simulink model "TJA1042_Loop_Example"  (R2024a)
(part 4 of 5)

      | CanConfigSet/CanController_0/CanCpuClockRef - /Mcu/Mcu/McuModuleConfiguration/McuClockSettingConfig_0/FLEXCAN_PE_CLK0_2 
      | CanConfigSet/CanController_0/CanCpuClockRefAlternate - /Mcu/Mcu/McuModuleConfiguration/McuClockSettingConfig_0/FLEXCAN_PE_CLK0_2 
      | CanConfigSet/CanController_0/CanHwChannel - FLEXCAN_0 
      | CanConfigSet/CanController_0/CanLoopBackMode - false 
      | CanConfigSet/CanController_0/CanRamBlock - CanRamBlock 
      | CanConfigSet/CanController_0/CanRamBlock/CanRamBlockUnified - CanRamBlockUnified 
      | CanConfigSet/CanController_0/CanRamBlock/CanRamBlockUnified/CanBlockUnifiedPayloadLength - CAN_16_BYTES_PAYLOAD 
      | CanConfigSet/CanController_0/CanRamBlock/Choice - CanRamBlockUnified 
      | CanConfigSet/CanController_0/CanRamBlock/Index - 0 
      | CanConfigSet/CanController_0/CanRxFiFo - CanRxFiFo 
      | CanConfigSet/CanController_0/CanRxFiFo/CanEnhanceFiFo - CanRxFiFo 
      | CanConfigSet/CanController_0/CanRxFiFo/CanRxFiFo/CanEnhanceFiFoDmaEnable - false 
      | CanConfigSet/CanController_0/CanRxFiFo/CanRxFiFo/CanEnhancedSchemeType - MASK_FILTER_SCHEME 
      | CanConfigSet/CanController_0/CanRxFiFo/CanRxFiFo/CanFiFoDmaErrorNotif - NULL_PTR 
      | CanConfigSet/CanController_0/CanRxFiFo/CanRxFiFo/CanFiFoOverflowNotif - MBDT_FlexCAN0_FifoOverflowNotif 
      | CanConfigSet/CanController_0/CanRxFiFo/CanRxFiFo/NumberMBTransferDMA - 1 
      | CanConfigSet/CanController_0/CanRxFiFo/Choice - CanEnhanceFiFo 
      | CanConfigSet/CanController_0/CanRxFiFo/Index - 0 
      | CanConfigSet/CanController_0/CanRxProcessing - MIXED 
      | CanConfigSet/CanController_0/CanTrippleSamplingEnable - false 
      | CanConfigSet/CanController_0/CanTxProcessing - MIXED 
      | CanConfigSet/CanController_0/CanWakeupFunctionalityAPI - false 
      | CanConfigSet/CanController_0/CanWakeupProcessing - POLLING 
      | CanConfigSet/CanController_0/CanWakeupSupport - false 
      | CanConfigSet/CanController_0/Index - 0 
      | CanConfigSet/CanController_1/CanAutoBusOffRecovery - false 
      | CanConfigSet/CanController_1/CanBusoffProcessing - POLLING 
      | CanConfigSet/CanController_1/CanControllerActivation - true 
      | CanConfigSet/CanController_1/CanControllerBaseAddress - 0 
      | CanConfigSet/CanController_1/CanControllerBaudrateConfig - CanControllerBaudrateConfig_0 
      | CanConfigSet/CanController_1/CanControllerBaudrateConfig_0/CanAdvancedSetting - false 
      | CanConfigSet/CanController_1/CanControllerBaudrateConfig_0/CanBaudrateTypeSuport - NORMAL_CBT 
      | CanConfigSet/CanController_1/CanControllerBaudrateConfig_0/CanBusLength - 40 
      | CanConfigSet/CanController_1/CanControllerBaudrateConfig_0/CanControllerBaudRate - 500.0 
      | CanConfigSet/CanController_1/CanControllerBaudrateConfig_0/CanControllerBaudRateConfigID - 0 
      | CanConfigSet/CanController_1/CanControllerBaudrateConfig_0/CanControllerPrescaller - 4 
      | CanConfigSet/CanController_1/CanControllerBaudrateConfig_0/CanControllerPrescallerAlternate - 10 
      | CanConfigSet/CanController_1/CanControllerBaudrateConfig_0/CanControllerPropSeg - 6 
      | CanConfigSet/CanController_1/CanControllerBaudrateConfig_0/CanControllerSeg1 - 8 
      | CanConfigSet/CanController_1/CanControllerBaudrateConfig_0/CanControllerSeg2 - 5 
      | CanConfigSet/CanController_1/CanControllerBaudrateConfig_0/CanControllerSyncJumpWidth - 4 
      | CanConfigSet/CanController_1/CanControllerBaudrateConfig_0/CanControllerSyncSeg - 1 
      | CanConfigSet/CanController_1/CanControllerBaudrateConfig_0/CanPropDelayTranceiver - 150.0 
      | CanConfigSet/CanController_1/CanControllerBaudrateConfig_0/CanTxArbitrationStartDelay - 12 
      | CanConfigSet/CanController_1/CanControllerBaudrateConfig_0/Index - 0 
      | CanConfigSet/CanController_1/CanControllerDefaultBaudrate - /Can_43_FLEXCAN/Can/CanConfigSet/CanController_1/CanControllerBaudrateConfig_0 
      | CanConfigSet/CanController_1/CanControllerEdgeFilter - false 
      | CanConfigSet/CanController_1/CanControllerFdISO - true 
      | CanConfigSet/CanController_1/CanControllerId - 1 
      | CanConfigSet/CanController_1/CanControllerPrExcEn - false 
      | CanConfigSet/CanController_1/CanCpuClockRef - /Mcu/Mcu/McuModuleConfiguration/McuClockSettingConfig_0/FLEXCAN_PE_CLK3_5 
      | CanConfigSet/CanController_1/CanCpuClockRefAlternate - /Mcu/Mcu/McuModuleConfiguration/McuClockSettingConfig_0/FLEXCAN_PE_CLK0_2 
      | CanConfigSet/CanController_1/CanHwChannel - FLEXCAN_4 
      | CanConfigSet/CanController_1/CanLoopBackMode - false 
      | CanConfigSet/CanController_1/CanRxFiFo - CanRxFiFo 
      | CanConfigSet/CanController_1/CanRxFiFo/CanLegacyFiFo - CanRxFiFo 
      | CanConfigSet/CanController_1/CanRxFiFo/CanRxFiFo/CanFiFoDmaErrorNotif - NULL_PTR 
      | CanConfigSet/CanController_1/CanRxFiFo/CanRxFiFo/CanFiFoOverflowNotif - MBDT_FlexCAN4_FifoOverflowNotif 
      | CanConfigSet/CanController_1/CanRxFiFo/CanRxFiFo/CanFiFoWarnNotif - MBDT_FlexCAN4_FifoWarnNotif 
      | CanConfigSet/CanController_1/CanRxFiFo/CanRxFiFo/CanIdAcceptanceMode - FORMAT_A 
      | CanConfigSet/CanController_1/CanRxFiFo/CanRxFiFo/CanLegacyFIFOGlobalMask0 - 0 
      | CanConfigSet/CanController_1/CanRxFiFo/CanRxFiFo/CanLegacyFIFOGlobalMask1 - 0 
      | CanConfigSet/CanController_1/CanRxFiFo/CanRxFiFo/CanLegacyFIFOGlobalMask2 - 0 
      | CanConfigSet/CanController_1/CanRxFiFo/CanRxFiFo/CanLegacyFIFOGlobalMask3 - 0 
      | CanConfigSet/CanController_1/CanRxFiFo/CanRxFiFo/CanLegacyFiFoDmaEnable - false 
      | CanConfigSet/CanController_1/CanRxFiFo/Choice - CanLegacyFiFo 
      | CanConfigSet/CanController_1/CanRxFiFo/Index - 0 
      | CanConfigSet/CanController_1/CanRxProcessing - MIXED 
      | CanConfigSet/CanController_1/CanTrippleSamplingEnable - false 
      | CanConfigSet/CanController_1/CanTxProcessing - MIXED 
      | CanConfigSet/CanController_1/CanWakeupFunctionalityAPI - false 
      | CanConfigSet/CanController_1/CanWakeupProcessing - POLLING 
      | CanConfigSet/CanController_1/CanWakeupSupport - false 
      | CanConfigSet/CanController_1/Index - 1 
      | CanConfigSet/CanHardwareObject - CanHardwareObject_Can0_Rx_Ext_Interrupt CanHardwareObject_Can0_Rx_FIFO CanHardwareObject_Can0_Rx_Std_Polling CanHardwareObject_Can0_Tx_Interrupt CanHardwareObject_Can0_Tx_Polling CanHardwareObject_Can4_Rx_Ext_Interrupt CanHardwareObject_Can4_Rx_FIFO CanHardwareObject_Can4_Rx_Std_Polling CanHardwareObject_Can4_Tx_Interrupt CanHardwareObject_Can4_Tx_Polling 
      | CanConfigSet/CanHardwareObject_Can0_Rx_Ext_Interrupt/CanControllerRef - /Can_43_FLEXCAN/Can/CanConfigSet/CanController_0 
      | CanConfigSet/CanHardwareObject_Can0_Rx_Ext_Interrupt/CanHandleType - BASIC 
      | CanConfigSet/CanHardwareObject_Can0_Rx_Ext_Interrupt/CanHardwareObjectUsesPolling - false 
      | CanConfigSet/CanHardwareObject_Can0_Rx_Ext_Interrupt/CanHwFilter - CanHwFilter_0 
      | CanConfigSet/CanHardwareObject_Can0_Rx_Ext_Interrupt/CanHwFilter_0/CanHwFilterCode - 0 
      | CanConfigSet/CanHardwareObject_Can0_Rx_Ext_Interrupt/CanHwFilter_0/CanHwFilterMask - 0 
      | CanConfigSet/CanHardwareObject_Can0_Rx_Ext_Interrupt/CanHwFilter_0/Index - 0 
      | CanConfigSet/CanHardwareObject_Can0_Rx_Ext_Interrupt/CanHwObjectCount - 1 
      | CanConfigSet/CanHardwareObject_Can0_Rx_Ext_Interrupt/CanIdType - EXTENDED 
      | CanConfigSet/CanHardwareObject_Can0_Rx_Ext_Interrupt/CanObjectId - 2 
      | CanConfigSet/CanHardwareObject_Can0_Rx_Ext_Interrupt/CanObjectType - RECEIVE 
      | CanConfigSet/CanHardwareObject_Can0_Rx_Ext_Interrupt/Index - 2 
      | CanConfigSet/CanHardwareObject_Can0_Rx_FIFO/CanControllerRef - /Can_43_FLEXCAN/Can/CanConfigSet/CanController_0 
      | CanConfigSet/CanHardwareObject_Can0_Rx_FIFO/CanHandleType - BASIC 
      | CanConfigSet/CanHardwareObject_Can0_Rx_FIFO/CanHardwareObjectUsesPolling - false 
      | CanConfigSet/CanHardwareObject_Can0_Rx_FIFO/CanHwFilter - CanHwFilter_0 CanHwFilter_1 CanHwFilter_2 CanHwFilter_3 CanHwFilter_4 CanHwFilter_5 CanHwFilter_6 CanHwFilter_7 
      | CanConfigSet/CanHardwareObject_Can0_Rx_FIFO/CanHwFilter_0/CanHwFilterCode - 1008 
      | CanConfigSet/CanHardwareObject_Can0_Rx_FIFO/CanHwFilter_0/CanHwFilterMask - 536870911 
      | CanConfigSet/CanHardwareObject_Can0_Rx_FIFO/CanHwFilter_0/Index - 0 
      | CanConfigSet/CanHardwareObject_Can0_Rx_FIFO/CanHwFilter_1/CanHwFilterCode - 1009 
      | CanConfigSet/CanHardwareObject_Can0_Rx_FIFO/CanHwFilter_1/CanHwFilterMask - 536870911 
      | CanConfigSet/CanHardwareObject_Can0_Rx_FIFO/CanHwFilter_1/Index - 1 
      | CanConfigSet/CanHardwareObject_Can0_Rx_FIFO/CanHwFilter_2/CanHwFilterCode - 1010 
      | CanConfigSet/CanHardwareObject_Can0_Rx_FIFO/CanHwFilter_2/CanHwFilterMask - 536870911 
      | CanConfigSet/CanHardwareObject_Can0_Rx_FIFO/CanHwFilter_2/Index - 2 
      | CanConfigSet/CanHardwareObject_Can0_Rx_FIFO/CanHwFilter_3/CanHwFilterCode - 1011 
      | CanConfigSet/CanHardwareObject_Can0_Rx_FIFO/CanHwFilter_3/CanHwFilterMask - 536870911 
      | CanConfigSet/CanHardwareObject_Can0_Rx_FIFO/CanHwFilter_3/Index - 3 
      | CanConfigSet/CanHardwareObject_Can0_Rx_FIFO/CanHwFilter_4/CanHwFilterCode - 1012 
      | CanConfigSet/CanHardwareObject_Can0_Rx_FIFO/CanHwFilter_4/CanHwFilterMask - 536870911 
      | CanConfigSet/CanHardwareObject_Can0_Rx_FIFO/CanHwFilter_4/Index - 4 
      | CanConfigSet/CanHardwareObject_Can0_Rx_FIFO/CanHwFilter_5/CanHwFilterCode - 1013 
      | CanConfigSet/CanHardwareObject_Can0_Rx_FIFO/CanHwFilter_5/CanHwFilterMask - 536870911 
      | CanConfigSet/CanHardwareObject_Can0_Rx_FIFO/CanHwFilter_5/Index - 5 
      | CanConfigSet/CanHardwareObject_Can0_Rx_FIFO/CanHwFilter_6/CanHwFilterCode - 1014 
      | CanConfigSet/CanHardwareObject_Can0_Rx_FIFO/CanHwFilter_6/CanHwFilterMask - 536870911 
      | CanConfigSet/CanHardwareObject_Can0_Rx_FIFO/CanHwFilter_6/Index - 6 
      | CanConfigSet/CanHardwareObject_Can0_Rx_FIFO/CanHwFilter_7/CanHwFilterCode - 1015 
      | CanConfigSet/CanHardwareObject_Can0_Rx_FIFO/CanHwFilter_7/CanHwFilterMask - 536870911 
      | CanConfigSet/CanHardwareObject_Can0_Rx_FIFO/CanHwFilter_7/Index - 7 
      | CanConfigSet/CanHardwareObject_Can0_Rx_FIFO/CanHwObjectCount - 6 
      | CanConfigSet/CanHardwareObject_Can0_Rx_FIFO/CanIdType - EXTENDED 
      | CanConfigSet/CanHardwareObject_Can0_Rx_FIFO/CanObjectId - 0 
      | CanConfigSet/CanHardwareObject_Can0_Rx_FIFO/CanObjectType - RECEIVE 
      | CanConfigSet/CanHardwareObject_Can0_Rx_FIFO/Index - 0 
      | CanConfigSet/CanHardwareObject_Can0_Rx_Std_Polling/CanControllerRef - /Can_43_FLEXCAN/Can/CanConfigSet/CanController_0 
      | CanConfigSet/CanHardwareObject_Can0_Rx_Std_Polling/CanHandleType - BASIC 
      | CanConfigSet/CanHardwareObject_Can0_Rx_Std_Polling/CanHardwareObjectUsesPolling - true 
      | CanConfigSet/CanHardwareObject_Can0_Rx_Std_Polling/CanHwFilter - CanHwFilter_0 
      | CanConfigSet/CanHardwareObject_Can0_Rx_Std_Polling/CanHwFilter_0/CanHwFilterCode - 0 
      | CanConfigSet/CanHardwareObject_Can0_Rx_Std_Polling/CanHwFilter_0/CanHwFilterMask - 0 
      | CanConfigSet/CanHardwareObject_Can0_Rx_Std_Polling/CanHwFilter_0/Index - 0 
      | CanConfigSet/CanHardwareObject_Can0_Rx_Std_Polling/CanHwObjectCount - 1 
      | CanConfigSet/CanHardwareObject_Can0_Rx_Std_Polling/CanIdType - STANDARD 
      | CanConfigSet/CanHardwareObject_Can0_Rx_Std_Polling/CanMainFunctionRWPeriodRef - /Can_43_FLEXCAN/Can/CanGeneral/CanMainFunctionRWPeriods_0 
      | CanConfigSet/CanHardwareObject_Can0_Rx_Std_Polling/CanObjectId - 1 
      | CanConfigSet/CanHardwareObject_Can0_Rx_Std_Polling/CanObjectType - RECEIVE 
      | CanConfigSet/CanHardwareObject_Can0_Rx_Std_Polling/Index - 1 
      | CanConfigSet/CanHardwareObject_Can0_Tx_Interrupt/CanControllerRef - /Can_43_FLEXCAN/Can/CanConfigSet/CanController_0 
      | CanConfigSet/CanHardwareObject_Can0_Tx_Interrupt/CanHandleType - BASIC 
      | CanConfigSet/CanHardwareObject_Can0_Tx_Interrupt/CanHardwareObjectUsesPolling - false 
      | CanConfigSet/CanHardwareObject_Can0_Tx_Interrupt/CanHwFilter - CanHwFilter_0 
      | CanConfigSet/CanHardwareObject_Can0_Tx_Interrupt/CanHwFilter_0/CanHwFilterCode - 0 
      | CanConfigSet/CanHardwareObject_Can0_Tx_Interrupt/CanHwFilter_0/CanHwFilterMask - 0 
      | CanConfigSet/CanHardwareObject_Can0_Tx_Interrupt/CanHwFilter_0/Index - 0 
      | CanConfigSet/CanHardwareObject_Can0_Tx_Interrupt/CanHwObjectCount - 1 
      | CanConfigSet/CanHardwareObject_Can0_Tx_Interrupt/CanIdType - MIXED 
      | CanConfigSet/CanHardwareObject_Can0_Tx_Interrupt/CanObjectId - 7 
      | CanConfigSet/CanHardwareObject_Can0_Tx_Interrupt/CanObjectType - TRANSMIT 
      | CanConfigSet/CanHardwareObject_Can0_Tx_Interrupt/Index - 7 
      | CanConfigSet/CanHardwareObject_Can0_Tx_Polling/CanControllerRef - /Can_43_FLEXCAN/Can/CanConfigSet/CanController_0 
      | CanConfigSet/CanHardwareObject_Can0_Tx_Polling/CanHandleType - BASIC 
      | CanConfigSet/CanHardwareObject_Can0_Tx_Polling/CanHardwareObjectUsesPolling - true 
      | CanConfigSet/CanHardwareObject_Can0_Tx_Polling/CanHwFilter - CanHwFilter_0 
      | CanConfigSet/CanHardwareObject_Can0_Tx_Polling/CanHwFilter_0/CanHwFilterCode - 0 
      | CanConfigSet/CanHardwareObject_Can0_Tx_Polling/CanHwFilter_0/CanHwFilterMask - 0 
      | CanConfigSet/CanHardwareObject_Can0_Tx_Polling/CanHwFilter_0/Index - 0 
      | CanConfigSet/CanHardwareObject_Can0_Tx_Polling/CanHwObjectCount - 1 
      | CanConfigSet/CanHardwareObject_Can0_Tx_Polling/CanIdType - MIXED 
      | CanConfigSet/CanHardwareObject_Can0_Tx_Polling/CanMainFunctionRWPeriodRef - /Can_43_FLEXCAN/Can/CanGeneral/CanMainFunctionRWPeriods_0 
      | CanConfigSet/CanHardwareObject_Can0_Tx_Polling/CanObjectId - 6 
      | CanConfigSet/CanHardwareObject_Can0_Tx_Polling/CanObjectType - TRANSMIT 
      | CanConfigSet/CanHardwareObject_Can0_Tx_Polling/Index - 6 
      | CanConfigSet/CanHardwareObject_Can4_Rx_Ext_Interrupt/CanControllerRef - /Can_43_FLEXCAN/Can/CanConfigSet/CanController_1 
      | CanConfigSet/CanHardwareObject_Can4_Rx_Ext_Interrupt/CanHandleType - BASIC 
      | CanConfigSet/CanHardwareObject_Can4_Rx_Ext_Interrupt/CanHardwareObjectUsesPolling - false 
      | CanConfigSet/CanHardwareObject_Can4_Rx_Ext_Interrupt/CanHwFilter - CanHwFilter_0 
      | CanConfigSet/CanHardwareObject_Can4_Rx_Ext_Interrupt/CanHwFilter_0/CanHwFilterCode - 0 
      | CanConfigSet/CanHardwareObject_Can4_Rx_Ext_Interrupt/CanHwFilter_0/CanHwFilterMask - 0 
      | CanConfigSet/CanHardwareObject_Can4_Rx_Ext_Interrupt/CanHwFilter_0/Index - 0 
      | CanConfigSet/CanHardwareObject_Can4_Rx_Ext_Interrupt/CanHwObjectCount - 1 
      | CanConfigSet/CanHardwareObject_Can4_Rx_Ext_Interrupt/CanIdType - EXTENDED 
      | CanConfigSet/CanHardwareObject_Can4_Rx_Ext_Interrupt/CanObjectId - 5 
      | CanConfigSet/CanHardwareObject_Can4_Rx_Ext_Interrupt/CanObjectType - RECEIVE 
      | CanConfigSet/CanHardwareObject_Can4_Rx_Ext_Interrupt/Index - 5 
      | CanConfigSet/CanHardwareObject_Can4_Rx_FIFO/CanControllerRef - /Can_43_FLEXCAN/Can/CanConfigSet/CanController_1 
      | CanConfigSet/CanHardwareObject_Can4_Rx_FIFO/CanHandleType - BASIC 
      | CanConfigSet/CanHardwareObject_Can4_Rx_FIFO/CanHardwareObjectUsesPolling - false 
      | CanConfigSet/CanHardwareObject_Can4_Rx_FIFO/CanHwFilter - CanHwFilter_0 CanHwFilter_1 CanHwFilter_2 CanHwFilter_3 CanHwFilter_4 CanHwFilter_5 CanHwFilter_6 CanHwFilter_7 
      | CanConfigSet/CanHardwareObject_Can4_Rx_FIFO/CanHwFilter_0/CanHwFilterCode - 1008 
      | CanConfigSet/CanHardwareObject_Can4_Rx_FIFO/CanHwFilter_0/CanHwFilterMask - 536870911 
      | CanConfigSet/CanHardwareObject_Can4_Rx_FIFO/CanHwFilter_0/Index - 0 
      | CanConfigSet/CanHardwareObject_Can4_Rx_FIFO/CanHwFilter_1/CanHwFilterCode - 1009 
      | CanConfigSet/CanHardwareObject_Can4_Rx_FIFO/CanHwFilter_1/CanHwFilterMask - 536870911 
      | CanConfigSet/CanHardwareObject_Can4_Rx_FIFO/CanHwFilter_1/Index - 1 
      | CanConfigSet/CanHardwareObject_Can4_Rx_FIFO/CanHwFilter_2/CanHwFilterCode - 1010 
      | CanConfigSet/CanHardwareObject_Can4_Rx_FIFO/CanHwFilter_2/CanHwFilterMask - 536870911 
      | CanConfigSet/CanHardwareObject_Can4_Rx_FIFO/CanHwFilter_2/Index - 2 
      | CanConfigSet/CanHardwareObject_Can4_Rx_FIFO/CanHwFilter_3/CanHwFilterCode - 1011 
      | CanConfigSet/CanHardwareObject_Can4_Rx_FIFO/CanHwFilter_3/CanHwFilterMask - 536870911 
      | CanConfigSet/CanHardwareObject_Can4_Rx_FIFO/CanHwFilter_3/Index - 3 
      | CanConfigSet/CanHardwareObject_Can4_Rx_FIFO/CanHwFilter_4/CanHwFilterCode - 1012 
      | CanConfigSet/CanHardwareObject_Can4_Rx_FIFO/CanHwFilter_4/CanHwFilterMask - 536870911 
      | CanConfigSet/CanHardwareObject_Can4_Rx_FIFO/CanHwFilter_4/Index - 4 
      | CanConfigSet/CanHardwareObject_Can4_Rx_FIFO/CanHwFilter_5/CanHwFilterCode - 1013 
      | CanConfigSet/CanHardwareObject_Can4_Rx_FIFO/CanHwFilter_5/CanHwFilterMask - 536870911 
      | CanConfigSet/CanHardwareObject_Can4_Rx_FIFO/CanHwFilter_5/Index - 5 
      | CanConfigSet/CanHardwareObject_Can4_Rx_FIFO/CanHwFilter_6/CanHwFilterCode - 1014 
      | CanConfigSet/CanHardwareObject_Can4_Rx_FIFO/CanHwFilter_6/CanHwFilterMask - 536870911 
      | CanConfigSet/CanHardwareObject_Can4_Rx_FIFO/CanHwFilter_6/Index - 6 
      | CanConfigSet/CanHardwareObject_Can4_Rx_FIFO/CanHwFilter_7/CanHwFilterCode - 1015 
      | CanConfigSet/CanHardwareObject_Can4_Rx_FIFO/CanHwFilter_7/CanHwFilterMask - 536870911 
      | CanConfigSet/CanHardwareObject_Can4_Rx_FIFO/CanHwFilter_7/Index - 7 
      | CanConfigSet/CanHardwareObject_Can4_Rx_FIFO/CanHwObjectCount - 6 
      | CanConfigSet/CanHardwareObject_Can4_Rx_FIFO/CanIdType - EXTENDED 
      | CanConfigSet/CanHardwareObject_Can4_Rx_FIFO/CanObjectId - 3 
      | CanConfigSet/CanHardwareObject_Can4_Rx_FIFO/CanObjectType - RECEIVE 
      | CanConfigSet/CanHardwareObject_Can4_Rx_FIFO/Index - 3 
      | CanConfigSet/CanHardwareObject_Can4_Rx_Std_Polling/CanControllerRef - /Can_43_FLEXCAN/Can/CanConfigSet/CanController_1 
      | CanConfigSet/CanHardwareObject_Can4_Rx_Std_Polling/CanHandleType - BASIC 
      | CanConfigSet/CanHardwareObject_Can4_Rx_Std_Polling/CanHardwareObjectUsesPolling - true 
      | CanConfigSet/CanHardwareObject_Can4_Rx_Std_Polling/CanHwFilter - CanHwFilter_0 
      | CanConfigSet/CanHardwareObject_Can4_Rx_Std_Polling/CanHwFilter_0/CanHwFilterCode - 0 
      | CanConfigSet/CanHardwareObject_Can4_Rx_Std_Polling/CanHwFilter_0/CanHwFilterMask - 0 
      | CanConfigSet/CanHardwareObject_Can4_Rx_Std_Polling/CanHwFilter_0/Index - 0 
      | CanConfigSet/CanHardwareObject_Can4_Rx_Std_Polling/CanHwObjectCount - 1 
      | CanConfigSet/CanHardwareObject_Can4_Rx_Std_Polling/CanIdType - STANDARD 
      | CanConfigSet/CanHardwareObject_Can4_Rx_Std_Polling/CanMainFunctionRWPeriodRef - /Can_43_FLEXCAN/Can/CanGeneral/CanMainFunctionRWPeriods_0 
      | CanConfigSet/CanHardwareObject_Can4_Rx_Std_Polling/CanObjectId - 4 
      | CanConfigSet/CanHardwareObject_Can4_Rx_Std_Polling/CanObjectType - RECEIVE 
      | CanConfigSet/CanHardwareObject_Can4_Rx_Std_Polling/Index - 4 
      | CanConfigSet/CanHardwareObject_Can4_Tx_Interrupt/CanControllerRef - /Can_43_FLEXCAN/Can/CanConfigSet/CanController_1 
      | CanConfigSet/CanHardwareObject_Can4_Tx_Interrupt/CanHandleType - BASIC 
      | CanConfigSet/CanHardwareObject_Can4_Tx_Interrupt/CanHardwareObjectUsesPolling - false 
      | CanConfigSet/CanHardwareObject_Can4_Tx_Interrupt/CanHwFilter - CanHwFilter_0 
      | CanConfigSet/CanHardwareObject_Can4_Tx_Interrupt/CanHwFilter_0/CanHwFilterCode - 0 
      | CanConfigSet/CanHardwareObject_Can4_Tx_Interrupt/CanHwFilter_0/CanHwFilterMask - 0 
      | CanConfigSet/CanHardwareObject_Can4_Tx_Interrupt/CanHwFilter_0/Index - 0 
      | CanConfigSet/CanHardwareObject_Can4_Tx_Interrupt/CanHwObjectCount - 1 
      | CanConfigSet/CanHardwareObject_Can4_Tx_Interrupt/CanIdType - MIXED 
      | CanConfigSet/CanHardwareObject_Can4_Tx_Interrupt/CanObjectId - 9 
      | CanConfigSet/CanHardwareObject_Can4_Tx_Interrupt/CanObjectType - TRANSMIT 
      | CanConfigSet/CanHardwareObject_Can4_Tx_Interrupt/Index - 9 
      | CanConfigSet/CanHardwareObject_Can4_Tx_Polling/CanControllerRef - /Can_43_FLEXCAN/Can/CanConfigSet/CanController_1 
      | CanConfigSet/CanHardwareObject_Can4_Tx_Polling/CanHandleType - BASIC 
      | CanConfigSet/CanHardwareObject_Can4_Tx_Polling/CanHardwareObjectUsesPolling - true 
      | CanConfigSet/CanHardwareObject_Can4_Tx_Polling/CanHwFilter - CanHwFilter_0 
      | CanConfigSet/CanHardwareObject_Can4_Tx_Polling/CanHwFilter_0/CanHwFilterCode - 0 
      | CanConfigSet/CanHardwareObject_Can4_Tx_Polling/CanHwFilter_0/CanHwFilterMask - 0 
      | CanConfigSet/CanHardwareObject_Can4_Tx_Polling/CanHwFilter_0/Index - 0 
      | CanConfigSet/CanHardwareObject_Can4_Tx_Polling/CanHwObjectCount - 1 
      | CanConfigSet/CanHardwareObject_Can4_Tx_Polling/CanIdType - MIXED 
      | CanConfigSet/CanHardwareObject_Can4_Tx_Polling/CanMainFunctionRWPeriodRef - /Can_43_FLEXCAN/Can/CanGeneral/CanMainFunctionRWPeriods_0 
      | CanConfigSet/CanHardwareObject_Can4_Tx_Polling/CanObjectId - 8 
      | CanConfigSet/CanHardwareObject_Can4_Tx_Polling/CanObjectType - TRANSMIT 
      | CanConfigSet/CanHardwareObject_Can4_Tx_Polling/Index - 8 
      | CanGeneral - CanGeneral 
      | CanGeneral/CanApiEnableMbAbort - true 
      | CanGeneral/CanDevErrorDetect - true 
      | CanGeneral/CanEnableDualClockMode - false 
      | CanGeneral/CanEnableSecurityEventReporting - false 
      | CanGeneral/CanEnableUserModeSupport - false 
      | CanGeneral/CanGlobalTimeSupport - false 
      | CanGeneral/CanIndex - 0 
      | CanGeneral/CanMBCountExtensionSupport - false 
      | CanGeneral/CanMainFunctionModePeriod - 0.001 
      | CanGeneral/CanMainFunctionRWPeriods - CanMainFunctionRWPeriods_0 
      | CanGeneral/CanMainFunctionRWPeriods_0/CanMainFunctionPeriod - 0.001 
      | CanGeneral/CanMainFunctionRWPeriods_0/Index - 0 
      | CanGeneral/CanMultiPartitionSupport - false 
      | CanGeneral/CanMultiplexedTransmission - true 
      | CanGeneral/CanSetBaudrateApi - true 
      | CanGeneral/CanTimeoutDuration - 1.0 
      | CanGeneral/CanTimeoutMethod - OSIF_COUNTER_DUMMY 
      | CanGeneral/CanVersionInfoApi - true 
      | CommonPublishedInformation - CommonPublishedInformation 
      | CommonPublishedInformation/ArReleaseMajorVersion - 4 
      | CommonPublishedInformation/ArReleaseMinorVersion - 7 
      | CommonPublishedInformation/ArReleaseRevisionVersion - 0 
      | CommonPublishedInformation/ModuleId - 80 
      | CommonPublishedInformation/SwMajorVersion - 3 
      | CommonPublishedInformation/SwMinorVersion - 0 
      | CommonPublishedInformation/SwPatchVersion - 0 
      | CommonPublishedInformation/VendorApiInfix - FLEXCAN 
      | CommonPublishedInformation/VendorId - 43 
      | IMPLEMENTATION-CONFIG-VARIANT - VARIANT-PRE-COMPILE 
      | POST_BUILD_VARIANT_USED - false
      settings: SourceProductName=Communication Blocks
  Data Store Write : DataStoreWrite  DataStoreName=SetControllerMode_Status  IndexOptions=Index vector (dialog)  Indices=1  OutputSizes=1
  Data Store Write1 : DataStoreWrite  DataStoreName=GetControllerMode_Status  IndexOptions=Index vector (dialog)  Indices=1  OutputSizes=1
  Data Store Write2 : DataStoreWrite  DataStoreName=GetControllerMode_Mode  IndexOptions=Index vector (dialog)  Indices=1  OutputSizes=1
  Data Store Write3 : DataStoreWrite  DataStoreName=GetControllerErrorState_Status  IndexOptions=Index vector (dialog)  Indices=1  OutputSizes=1
  Data Store Write4 : DataStoreWrite  DataStoreName=GetControllerErrorState_State  IndexOptions=Index vector (dialog)  Indices=1  OutputSizes=1
  Data Store Write5 : DataStoreWrite  DataStoreName=GetVersionInfo_VersionInfo  IndexOptions=Index vector (dialog)  Indices=1  OutputSizes=1
  Event Listener : EventListener  DisableCoverage=on  EventName=reset
  wires:
  Can_SetControllerMode/1 -> Data Store Write/1
  Can_GetControllerMode/1 -> Data Store Write1/1
  Can_GetControllerMode/2 -> Data Store Write2/1
  Can_GetControllerErrorState/2 -> Data Store Write4/1
  Can_GetControllerErrorState/1 -> Data Store Write3/1
  Can_GetVersionInfo/1 -> Data Store Write5/1
